simulink model "s_cd_hmc_v2"  (R2016b)
(part 14 of 43)

  Relational5/1 -> Delay3/1, Register10/2, Register4/2, Delay5/1
  Counter9/1 -> Register10/1
  Counter7/1 -> Register4/1
  pipeline155/1(q) -> data_out_counter/1(out_counter)
  pipeline156/1(q) -> data_in_counter/1(out_counter)
  Counter6/1 -> Relational5/1
  pipeline159/1(q) -> Gateway Out3/1, [radd]
  pipeline162/1(q) -> Gateway Out91/1, [din]
  pipeline163/1(q) -> Delay81/1
  [hmc_dvalid] -> Reorder_cntrl/3(dvalid)
  pipeline167/1(q) -> Gateway Out46/1, hmc/7
  pipeline168/1(q) -> Gateway Out47/1, hmc/8
  pipeline169/1(q) -> Gateway Out49/1, hmc/9
  pipeline170/1(q) -> Gateway Out51/1, hmc/10
  pipeline171/1(q) -> Gateway Out52/1, hmc/11
  pipeline172/1(q) -> Gateway Out53/1, hmc/12
  bus_expand12/1(msb_out8) -> Gateway Out40/1
  bus_expand12/5(out4) -> Gateway Out61/1
  bus_expand12/6(out3) -> Gateway Out62/1
  bus_expand12/7(out2) -> Gateway Out63/1
  bus_expand12/4(out5) -> Gateway Out60/1
  bus_expand12/3(out6) -> Gateway Out44/1
  bus_expand12/2(out7) -> Gateway Out41/1
  bus_expand12/8(lsb_out1) -> Gateway Out64/1
  bus_expand11/1(msb_out8) -> Gateway Out65/1
  bus_expand11/2(out7) -> Gateway Out66/1
  bus_expand11/3(out6) -> Gateway Out67/1
  bus_expand11/4(out5) -> Gateway Out68/1
  bus_expand11/5(out4) -> Gateway Out69/1
  bus_expand11/6(out3) -> Gateway Out70/1
  bus_expand11/7(out2) -> Gateway Out71/1
  bus_expand11/8(lsb_out1) -> Gateway Out72/1
  Gateway Out72/1 -> To Workspace66/1
  Gateway Out71/1 -> To Workspace65/1
  Gateway Out70/1 -> To Workspace64/1
  Gateway Out69/1 -> To Workspace63/1
  Gateway Out68/1 -> To Workspace62/1
  Gateway Out67/1 -> To Workspace61/1
  Gateway Out66/1 -> To Workspace35/1
  Gateway Out65/1 -> To Workspace60/1
  Gateway Out63/1 -> To Workspace58/1
  Gateway Out64/1 -> To Workspace59/1
  Gateway Out62/1 -> To Workspace57/1
  Gateway Out61/1 -> To Workspace56/1
  Gateway Out60/1 -> To Workspace55/1
  Gateway Out44/1 -> To Workspace54/1
  Gateway Out41/1 -> To Workspace53/1
  Gateway Out40/1 -> To Workspace34/1
  bus_expand13/2(out7) -> Gateway Out73/1
  bus_expand13/3(out6) -> Gateway Out74/1
  bus_expand13/4(out5) -> Gateway Out75/1
  bus_expand13/5(out4) -> Gateway Out76/1
  bus_expand13/6(out3) -> Gateway Out77/1
  bus_expand13/7(out2) -> Gateway Out78/1
  bus_expand13/8(lsb_out1) -> Gateway Out79/1
  Gateway Out79/1 -> To Workspace74/1
  Gateway Out78/1 -> To Workspace73/1
  Gateway Out77/1 -> To Workspace72/1
  Gateway Out76/1 -> To Workspace71/1
  Gateway Out75/1 -> To Workspace70/1
  Gateway Out74/1 -> To Workspace69/1
  Gateway Out73/1 -> To Workspace67/1
  [q_out] -> bus_expand13/1(bus_in)
  bus_expand13/1(msb_out8) -> Gateway Out80/1
  Gateway Out80/1 -> To Workspace68/1
  [hmc_reord_dvalid] -> FIFO1/2, Gateway Out16/1
  bus_expand1/1(msb_out8) -> pipeline37/1(d)  "hmc_out1"
  bus_expand1/8(lsb_out1) -> pipeline44/1(d)  "hmc_out8"
  [fifo1_dout] -> pipeline49/1(d)
  bus_expand2/1(msb_out8) -> pipeline26/1(d)  "hmc_out9"
  bus_expand2/8(lsb_out1) -> pipeline36/1(d)  "hmc_out16"
  [fifo0_dout] -> pipeline71/1(d)
  pipeline37/1(q) -> fifo1/1(in_d00)
  pipeline38/1(q) -> fifo1/2(in_d01)
  pipeline39/1(q) -> fifo1/3(in_d02)
  pipeline41/1(q) -> fifo1/5(in_d04)
  pipeline42/1(q) -> fifo1/6(in_d05)
  pipeline43/1(q) -> fifo1/7(in_d06)
  pipeline36/1(q) -> fifo0/8(in_d07)
  pipeline35/1(q) -> fifo0/7(in_d06)
  pipeline34/1(q) -> fifo0/6(in_d05)
  pipeline33/1(q) -> fifo0/5(in_d04)
  pipeline32/1(q) -> fifo0/4(in_d03)
  pipeline31/1(q) -> fifo0/3(in_d02)
  pipeline30/1(q) -> fifo0/2(in_d01)
  pipeline26/1(q) -> fifo0/1(in_d00)
  bus_expand1/2(out7) -> pipeline38/1(d)
  bus_expand1/4(out5) -> pipeline40/1(d)
  bus_expand1/7(out2) -> pipeline43/1(d)
  bus_expand1/3(out6) -> pipeline39/1(d)
  bus_expand2/7(out2) -> pipeline35/1(d)
  bus_expand1/5(out4) -> pipeline41/1(d)
  bus_expand1/6(out3) -> pipeline42/1(d)
  bus_expand2/5(out4) -> pipeline33/1(d)
  bus_expand2/4(out5) -> pipeline32/1(d)
  bus_expand2/6(out3) -> pipeline34/1(d)
  bus_expand2/3(out6) -> pipeline31/1(d)
  bus_expand2/2(out7) -> pipeline30/1(d)
  Convert28/1 -> pipeline45/1(d)
  pipeline44/1(q) -> fifo1/8(in_d07)
  pipeline40/1(q) -> fifo1/4(in_d03)
  Convert22/1 -> pipeline57/1(d)
  [hmc_reord_sync] -> pipeline52/1(d)
  pipeline56/1(q) -> fifo0/17(trig)
  pipeline57/1(q) -> fifo0/16(we)
  pipeline59/1(q) -> fifo0/10(in_per_full)
  pipeline58/1(q) -> fifo0/11(in_full)
  pipeline60/1(q) -> fifo0/9(in_empty)
  FIFO0/3 -> [fifo0_per_full]
  [fifo0_empty] -> pipeline64/1(d)
  [fifo0_per_full] -> pipeline63/1(d)
  [fifo0_full] -> pipeline62/1(d)
  FIFO1/3 -> [fifo1_per_full]
  [fifo0_dout] -> bus_expand12/1(bus_in)
  [fifo1_dout] -> bus_expand11/1(bus_in)
  [mux_sel] -> Gateway Out18/1, Mux/1
  pipeline45/1(q) -> fifo1/16(we)
  pipeline46/1(q) -> fifo1/17(trig)
  pipeline65/1(q) -> fifo1/9(in_empty)
  pipeline66/1(q) -> fifo1/10(in_per_full)
  pipeline67/1(q) -> fifo1/11(in_full)
  [fifo1_full] -> pipeline68/1(d)
  [fifo1_per_full] -> pipeline51/1(d)
  [fifo1_empty] -> pipeline50/1(d)
  [mux_sel] -> pipeline55/1(d)
  pipeline72/1(q) -> fifo0/12(in_mux_sel)
  pipeline73/1(q) -> fifo1/12(in_mux_sel)
  [mux_sel] -> pipeline69/1(d)
  [hmc_reord_dvalid] -> FIFO0/2, Gateway Out12/1
  Logical18/1 -> Gateway Out120/1, Delay7/1, edge_detect11/1(in)
  Convert19/1 -> Gateway Out45/1, Logical2/2
  [fifo0_dout] -> Slice11/1
  [fifo1_dout] -> Slice3/1
  Convert17/1 -> Gateway Out43/1, Logical2/1
  Counter/1 -> Convert12/1, Convert14/1
  Logical21/1 -> Gateway Out145/1, edge_detect10/1(in)
  Logical23/1 -> Gateway Out146/1, edge_detect28/1(in)
  Inverter7/1 -> Gateway Out148/1, Logical21/2
  Inverter8/1 -> Gateway Out147/1, Logical23/2
  [fifo1_re] -> FIFO1/3, Gateway Out17/1
  Convert15/1 -> Gateway Out149/1, Logical23/1
  hmc_delay/1(sim_out) -> To Workspace5/1
  [hmc_delay] -> Convert4/1
  Convert4/1 -> hmc_delay/1(out_delay)
  [hmc_sync] -> Reorder_cntrl/1(rst)
  Gateway Out22/1 -> To Workspace9/1
  Slice8/1 -> bus_expand4/1(bus_in)
  [hmc_reord_data] -> Slice8/1
  bus_expand4/1(msb_out8) -> Gateway Out22/1
  Gateway Out24/1 -> To Workspace11/1
  Gateway Out25/1 -> To Workspace18/1
  Gateway Out26/1 -> To Workspace19/1
  bus_expand4/4(out5) -> Gateway Out26/1
  bus_expand4/3(out6) -> Gateway Out25/1
  bus_expand4/2(out7) -> Gateway Out24/1
  Gateway Out27/1 -> To Workspace21/1
  bus_expand4/5(out4) -> Gateway Out27/1
  Gateway Out28/1 -> To Workspace22/1
  bus_expand4/6(out3) -> Gateway Out28/1
  Gateway Out29/1 -> To Workspace23/1
  bus_expand4/7(out2) -> Gateway Out29/1
  Gateway Out30/1 -> To Workspace24/1
  bus_expand4/8(lsb_out1) -> Gateway Out30/1
  Slice10/1 -> bus_expand6/1(bus_in)
  [hmc_reord_data] -> Slice10/1
  Gateway Out31/1 -> To Workspace77/1
  Gateway Out32/1 -> To Workspace27/1
  Gateway Out33/1 -> To Workspace28/1
  Gateway Out35/1 -> To Workspace29/1
  Gateway Out37/1 -> To Workspace31/1
  Gateway Out38/1 -> To Workspace32/1
  Gateway Out39/1 -> To Workspace33/1
  Gateway Out42/1 -> To Workspace36/1
  bus_expand6/1(msb_out8) -> Gateway Out31/1
  bus_expand6/2(out7) -> Gateway Out32/1
  bus_expand6/3(out6) -> Gateway Out33/1
  bus_expand6/4(out5) -> Gateway Out35/1
  bus_expand6/5(out4) -> Gateway Out37/1
  bus_expand6/6(out3) -> Gateway Out38/1
  bus_expand6/7(out2) -> Gateway Out39/1
  bus_expand6/8(lsb_out1) -> Gateway Out42/1
  Gateway Out99/1 -> To Workspace94/1
  Gateway Out100/1 -> To Workspace95/1
  Gateway Out101/1 -> To Workspace96/1
  Gateway Out102/1 -> To Workspace97/1
  Gateway Out103/1 -> To Workspace98/1
  cd_hmc_sync_in/1(sim_out) -> To Workspace102/1
  cd_hmc_sync_out/1(sim_out) -> To Workspace101/1
  pipeline81/1(q) -> Register1/3, Register1/1
  pipeline82/1(q) -> Register5/3, Register5/1
  Register5/1 -> pipeline132/1(d)
  pipeline102/1(q) -> Register1/2
  pipeline108/1(q) -> Register5/2
  cd_hmc_sync_in_cnt/1(sim_out) -> To Workspace104/1
  Counter10/1 -> pipeline129/1(d)
  cd_hmc_sync_out_cnt/1(sim_out) -> To Workspace105/1
  Counter11/1 -> pipeline113/1(d)
  pipeline113/1(q) -> cd_hmc_sync_out_cnt/1(out_reg)
  pipeline129/1(q) -> cd_hmc_sync_in_cnt/1(out_reg)
  pipeline131/1(q) -> cd_hmc_sync_in/1(out_reg)
  pipeline132/1(q) -> cd_hmc_sync_out/1(out_reg)
  pipeline146/1(q) -> cd_hmc_rd_tag_err_count/1(out_counter)
  pipeline147/1(q) -> cd_hmc_fifo_full/1(out_full)
  pipeline148/1(q) -> cd_hmc_fifo_empty/1(out_empty)
  [fifo1_per_full] -> pipeline14/1(d)
  pipeline165/1(q) -> cd_hmc_rd_tag_err/1(out_error)
  Register1/1 -> pipeline131/1(d)
  sync_mon_rst/1(in_reg) -> pipeline98/1(d)
  Constant18/1 -> sync_mon_rst/1(sim_1)
  pipeline91/1(q) -> Counter11/1
  pipeline110/1(q) -> Counter11/2
  pipeline90/1(q) -> Counter10/1
  pipeline109/1(q) -> Counter10/2
  Gateway Out19/1 -> To Workspace4/1
  pipeline3/1(q) -> hmc/2, Gateway Out99/1  "hmc_wadd"
  hmc/1 -> Slice42/1, Slice43/1, pipeline19/1(d), Slice6/1, Slice13/1
  Slice13/1 -> Convert16/1
  Gateway Out87/1 -> To Workspace82/1
  [hmc_win_p0] -> pipeline173/1(d)
  Gateway Out90/1 -> To Workspace85/1
  read_tag_check/1(rd_tag_err) -> pipeline165/1(d)
  read_tag_check/2(rd_tag_err_count) -> pipeline146/1(d)
  cd_hmc_wr_req_count/1(sim_out) -> To Workspace115/1
  Counter3/1 -> pipeline4/1(d)
  pipeline4/1(q) -> cd_hmc_wr_req_count/1(out_reg)
  pipeline18/1(q) -> Counter3/1
  pipeline166/1(q) -> Counter3/2
  cd_hmc_rd_req_count/1(sim_out) -> To Workspace116/1
  Counter12/1 -> pipeline177/1(d)
  pipeline177/1(q) -> cd_hmc_rd_req_count/1(out_reg)
  pipeline176/1(q) -> Counter12/1
  pipeline175/1(q) -> Counter12/2
  [hmc_dvalid] -> pipeline183/1(d)  "tp2"
  [hmc_tag_out] -> pipeline180/1(d)  "tp1"
  [hmc_tag_pol0] -> pipeline181/1(d)
  [hmc_sync] -> pipeline182/1(d)
  pipeline181/1(q) -> read_tag_check/1(HMC_tag_in)
  pipeline180/1(q) -> read_tag_check/2(HMC_tag_out)
  pipeline183/1(q) -> read_tag_check/3(HMC_dvalid)
  pipeline182/1(q) -> read_tag_check/4(HMC_sync)
  cd_hmc_rd_dvalid_count/1(sim_out) -> To Workspace119/1
  Counter13/1 -> pipeline186/1(d)
  pipeline186/1(q) -> cd_hmc_rd_dvalid_count/1(out_reg)
  pipeline185/1(q) -> Counter13/1
  pipeline184/1(q) -> Counter13/2
  Constant20/1 -> dvalid_capture_cntrl/1(sim_1)
  dvalid_capture_cntrl/1(in_reg) -> pipeline78/1(d)
  Logical15/1 -> pipeline184/1(d)
  [hmc_dvalid] -> pipeline220/1(d)
  Logical/1 -> pipeline175/1(d)
  [hmc_rin_pol0] -> pipeline217/1(d)
  Logical16/1 -> pipeline166/1(d)
  [hmc_win_pol0] -> pipeline214/1(d)
  pipeline76/1(q) -> Logical16/1
  pipeline77/1(q) -> Logical/1
  pipeline75/1(q) -> Logical15/1
  pipeline78/1(q) -> [capture_cntrl]
  [capture_cntrl] -> pipeline75/1(d)
  [capture_cntrl] -> pipeline77/1(d)
  [capture_cntrl] -> pipeline76/1(d)
  pipeline83/1(q) -> read_tag_check/5(Capture_cntrl)
  [capture_cntrl] -> pipeline83/1(d)
  pipeline213/1(q) -> pipeline18/1(d)
  Logical30/1 -> pipeline185/1(d)
  pipeline216/1(q) -> pipeline176/1(d)
  [hmc_sync] -> pipeline218/1(d)
  Constant22/1 -> dvalid_capture_cntrl_rst/1(sim_1)
  dvalid_capture_cntrl_rst/1(in_reg) -> pipeline84/1(d)
  pipeline84/1(q) -> edge_detect16/1
  [capture_cntrl_rst] -> pipeline216/1(d)
  [capture_cntrl_rst] -> pipeline219/1(d)
  [capture_cntrl_rst] -> pipeline213/1(d)
  cd_reord_sync_out/1(sim_out) -> To Workspace117/1
  Register12/1 -> pipeline85/1(d)
  [sync_mon_rst] -> edge_detect1/1
  pipeline85/1(q) -> cd_reord_sync_out/1(out_reg)
  pipeline86/1(q) -> Register12/3, Register12/1
  [sync_mon_rst] -> edge_detect31/1
  pipeline98/1(q) -> [sync_mon_rst]
  cd_reord_sync_cnt/1(sim_out) -> To Workspace118/1
  Counter14/1 -> pipeline88/1(d)
  pipeline88/1(q) -> cd_reord_sync_cnt/1(out_reg)
  pipeline87/1(q) -> Counter14/2
  pipeline92/1(q) -> Register12/2
  pipeline89/1(q) -> Counter14/1
  [hmc_rin_p0] -> pipeline17/1(d)
  [hmc_raddr_p0] -> pipeline5/1(d)
  [hmc_tag_p0] -> pipeline16/1(d)
  cd_hmc_sync/1(sim_out) -> To Workspace112/1
  Counter15/1 -> pipeline95/1(d)
  pipeline95/1(q) -> cd_hmc_sync/1(out_reg)
  pipeline94/1(q) -> Counter15/1
  pipeline93/1(q) -> Counter15/2
  [hmc_sync] -> pipeline211/1(d)
  [sync_mon_rst] -> pipeline210/1(d)
  pipeline210/1(q) -> edge_detect23/1
  pipeline211/1(q) -> edge_detect17/1
  Logical35/1 -> Counter1/2, Gateway Out8/1
  [hmc_dout] -> HMC_reord_bram/2, Gateway Out11/1, Slice33/1, Slice32/1
  Gateway Out98/1 -> To Workspace100/1
  Gateway Out105/1 -> To Workspace109/1
  hmc/2 -> Logical34/2, pipeline20/1(d), Gateway Out105/1
  [wadd] -> hmc_control/1(waddr)
  [hmc_delay] -> hmc_control/2(delay)
  [hmc_sync] -> hmc_control/3(sync_in)
  [win] -> hmc_control/4(win)
  [rin] -> hmc_control/5(rin)
  [radd] -> hmc_control/6(rdadd)
  [din] -> hmc_control/7(din)
  hmc_control/3(hmc_rin) -> [hmc_rin_pol0]
  hmc_control/4(hmc_raddr) -> [hmc_raddr_pol0]
  hmc_control/6(hmc_tag) -> [hmc_tag_pol0]
  [hmc_rin_pol0] -> pipeline198/1(d)
  [hmc_tag_out] -> pipeline193/1(d)
  [hmc_tag_pol0] -> pipeline196/1(d)
  [hmc_raddr_pol0] -> pipeline197/1(d)
  [hmc_rd_rdy] -> pipeline194/1(d)
  [hmc_dvalid] -> pipeline195/1(d)
  pipeline6/1(q) -> hmc_debug0_p0/4(in_rin)
  pipeline7/1(q) -> hmc_debug0_p0/5(in_rdaddr)
  pipeline8/1(q) -> hmc_debug0_p0/6(in_tag_in)
  pipeline96/1(q) -> hmc_debug0_p0/7(in_dvalid)
  pipeline99/1(q) -> hmc_debug0_p0/8(in_rd_rdy)
  pipeline100/1(q) -> hmc_debug0_p0/9(in_tag_out)
  pipeline178/1(q) -> Gateway Out57/1, hmc_debug0_p0/10(we)
  [hmc_tag_out] -> pipeline188/1(d)
  [hmc_rd_rdy] -> pipeline189/1(d)
  [hmc_dvalid] -> pipeline190/1(d)
  pipeline191/1(q) -> hmc_debug1_p0/1(in_dvalid)
  pipeline192/1(q) -> hmc_debug1_p0/2(in_rd_rdy)
  pipeline179/1(q) -> hmc_debug1_p0/3(in_tag_out)
  pipeline187/1(q) -> hmc_debug1_p0/4(we)
  pipeline188/1(q) -> pipeline179/1(d)
  pipeline189/1(q) -> pipeline192/1(d)
  pipeline190/1(q) -> pipeline191/1(d)
  pipeline193/1(q) -> pipeline100/1(d)
  pipeline194/1(q) -> pipeline99/1(d)
  pipeline195/1(q) -> pipeline96/1(d)
  pipeline196/1(q) -> pipeline8/1(d)
  pipeline197/1(q) -> pipeline7/1(d)
  pipeline198/1(q) -> pipeline6/1(d)
  pipeline199/1(q) -> [rin], Gateway Out4/1
  [hmc_wr_ready] -> pipeline200/1(d)
  pipeline200/1(q) -> pipeline201/1(d)
  pipeline201/1(q) -> hmc_debug0_p0/2(in_wr_rdy)
  [hmc_win_pol0] -> pipeline203/1(d)
  [hmc_waddr_pol0] -> pipeline202/1(d)
  pipeline202/1(q) -> pipeline204/1(d)
  pipeline203/1(q) -> pipeline205/1(d)
  pipeline204/1(q) -> Gateway Out58/1, hmc_debug0_p0/3(in_waddr)
  pipeline205/1(q) -> Gateway Out59/1, hmc_debug0_p0/1(in_win)
  Delay28/1 -> Delay31/1
  Gateway Out1/1 -> To Workspace6/1
  Gateway Out2/1 -> To Workspace7/1
  Gateway Out3/1 -> To Workspace8/1
  Gateway Out4/1 -> To Workspace20/1
  Convert2/1 -> Delay22/1, addr/2
  pipeline214/1(q) -> Logical16/2
  pipeline217/1(q) -> Logical/2
  pipeline218/1(q) -> Logical30/1
  pipeline219/1(q) -> Logical30/2
  pipeline220/1(q) -> Logical15/2
  Logical24/1 -> addr/1, addr_stall/1
  pipeline13/1(q) -> Logical24/1
  pipeline9/1(q) -> Logical27/1
  edge_detect24/1(out) -> Logical24/2
  pipeline2/1(q) -> [hmc_delay]
  pipeline206/1(q) -> [dout]
  pipeline12/1(q) -> Delay23/1
  pipeline157/1(q) -> Gateway Out86/1, hmc_debug0_p0/11(trig)
  Logical32/1 -> edge_detect13/1(in)
  Logical29/1 -> edge_detect5/1(in)
  pipeline158/1(q) -> hmc_debug1_p0/5(trig)
  Delay36/1 -> Delay33/1
  pipeline23/1(q) -> [hmc_rd_rdy]  "rd_ready"
  AddSub/1 -> Delay32/1  "rd_add_HR"
  Gateway Out5/1 -> To Workspace30/1
  Gateway Out6/1 -> To Workspace75/1
  Reorder_cntrl/1(bram_rd_addr) -> Gateway Out6/1, HMC_reord_bram/4
  Gateway Out7/1 -> To Workspace76/1
  [hmc_tag_out] -> Reorder_cntrl/2(tag)
  Gateway Out13/1 -> To Workspace84/1
  Gateway Out11/1 -> To Workspace81/1
  pipeline209/1(q) -> [hmc_sync], Gateway Out19/1
  Slice18/1 -> Convert20/1
  [hmc_dvalid] -> Gateway Out13/1, HMC_reord_bram/3
  Convert1/1 -> [hmc_dvalid]
  pipeline1/1(q) -> Delay37/1
  pipeline79/1(q) -> [q_dvalid], Gateway Out84/1, dv/1
  Slice19/1 -> Convert21/1
  [hmc_sync] -> Counter1/1
  edge_detect11/1(out) -> Gateway Out142/1
  Logical4/1 -> Convert15/1
  Inverter1/1 -> Gateway Out150/1, Logical4/1
  Delay7/1 -> Counter/2, Gateway Out143/1, Logical4/2
  Convert12/1 -> Inverter1/1
  hmc_wr_err/1(sim_out) -> To Workspace136/1
  Counter16/1 -> pipeline10/1(d)
  pipeline10/1(q) -> hmc_wr_err/1(out_reg)
  pipeline223/1(q) -> Counter16/1
  [sync_mon_rst] -> edge_detect26/1
  [hmc_wr_ready] -> Inverter/1
  Inverter/1 -> Logical5/1
  pipeline224/1(q) -> Counter16/2
  Logical5/1 -> pipeline224/1(d)
  hmc_rd_err/1(sim_out) -> To Workspace137/1
  Counter17/1 -> pipeline225/1(d)
  pipeline225/1(q) -> hmc_rd_err/1(out_reg)
  pipeline226/1(q) -> Counter17/1
  [sync_mon_rst] -> edge_detect15/1
  [hmc_rd_rdy] -> Inverter12/1
  Inverter12/1 -> Logical6/1
  pipeline227/1(q) -> Counter17/2
  Logical6/1 -> pipeline227/1(d)
  [hmc_rd_rdy] -> Logical31/1
  Logical31/1 -> edge_detect24/1(in), Logical27/2
  Delay33/1 -> pipeline209/1(d)
  Delay32/1 -> pipeline159/1(d)
  Delay31/1 -> pipeline232/1(d), pipeline199/1(d)
  Delay25/1 -> pipeline162/1(d)
  [hmc_reord_data] -> Slice17/1
  [hmc_reord_data] -> Slice20/1
  Slice21/1 -> Convert17/1
  Slice22/1 -> Convert19/1
  [fifo0_dout] -> Slice21/1
  [fifo1_dout] -> Slice22/1
  Gateway Out8/1 -> To Workspace78/1
  Gateway Out9/1 -> To Workspace79/1
  Gateway Out10/1 -> To Workspace80/1
  Gateway Out12/1 -> To Workspace83/1
  Gateway Out14/1 -> To Workspace86/1
  [fifo0_re] -> FIFO0/3, Gateway Out14/1
  Gateway Out15/1 -> To Workspace87/1
  Gateway Out16/1 -> To Workspace88/1
  Gateway Out17/1 -> To Workspace89/1
  Gateway Out20/1 -> To Workspace91/1
  Gateway Out21/1 -> To Workspace92/1
  [hmc_reord_sync] -> pipeline86/1(d), pipeline87/1(d)
  Gateway Out18/1 -> To Workspace90/1
  Gateway Out36/1 -> To Workspace106/1
  Gateway Out81/1 -> To Workspace107/1
  Slice24/1 -> Convert23/1
  Convert24/1 -> Logical33/2
  Convert23/1 -> Logical33/1
  Slice25/1 -> Convert24/1
  Logical33/1 -> Convert25/1
  Convert25/1 -> edge_detect32/1
  [fifo_sync] -> delay1/1  "sync"
  Gateway Out82/1 -> To Workspace108/1
  HMC_reord_bram/2 -> Delay2/1, Slice25/1, Slice24/1, Slice18/1, Slice19/1
  Gateway Out23/1 -> To Workspace93/1
  Gateway Out34/1 -> To Workspace99/1
  Gateway Out83/1 -> To Workspace110/1
  Gateway Out84/1 -> To Workspace111/1
  Gateway Out85/1 -> To Workspace113/1
  [fifo_dvalid] -> delay8/1
  Counter19/1 -> Convert29/1
  Convert29/1 -> [mux_sel]
  [hmc_sync] -> Counter19/1
  Gateway Out43/1 -> To Workspace37/1
  Gateway Out45/1 -> To Workspace38/1
  Logical27/1 -> addr_stall/2
  misci/1 -> Gateway Out138/1, Slice29/1, Delay21/1
  [sync_in] -> pipeline1/1(d), pipeline13/1(d)
  [en_in] -> pipeline9/1(d), pipeline12/1(d)
  en/1 -> Gateway Out140/1, [en_in]  "en_in"
  Delay70/1 -> pipeline233/1(d)
  AddSub2/1 -> AddSub/2
  Constant/1 -> AddSub2/2
  [delay_in] -> AddSub2/1
  Slice29/1 -> [ld_val]
  pipeline232/1(q) -> Gateway Out2/1, [win]
  [hmc_tag_out] -> Gateway Out5/1, HMC_reord_bram/1
  [ld_val] -> Register13/2
  delay/1 -> Register13/1  "delay"
  Register13/1 -> [delay_in], pipeline2/1(d)
  hmc_wr_rd_rdy_clash/1(sim_out) -> To Workspace124/1
  Counter20/1 -> pipeline207/1(d)
  pipeline207/1(q) -> hmc_wr_rd_rdy_clash/1(out_reg)
  pipeline208/1(q) -> Counter20/1
  pipeline231/1(q) -> Counter20/2
  [sync_mon_rst] -> edge_detect14/1
  [hmc_rd_rdy] -> Logical19/2
  [hmc_wr_ready] -> Logical19/1
  Logical19/1 -> pipeline231/1(d)
  Gateway Out91/1 -> To Workspace125/1
  Gateway Out93/1 -> To Workspace126/1
  delay2/1 -> Terminator1/1, Gateway Out34/1
  Gateway Out106/1 -> To Workspace132/1
  Gateway Out107/1 -> To Workspace133/1
  Gateway Out108/1 -> To Workspace134/1
  pipeline233/1(q) -> Gateway Out1/1, [wadd]
  Delay1/1 -> Delay70/1
  delay1/1 -> pipeline117/1(d), Gateway Out108/1
  delay8/1 -> pipeline79/1(d), Gateway Out107/1
  Slice5/1 -> Convert7/1
  Gateway Out121/1 -> To Workspace150/1
  Convert7/1 -> Gateway Out121/1
  Convert20/1 -> Logical35/1
  Convert21/1 -> Logical35/2
  Delay2/1 -> Gateway Out93/1, [hmc_reord_data]
  Convert8/1 -> [hmc_reord_dvalid], Gateway Out9/1
  [hmc_waddr_p0] -> pipeline3/1(d)
  Gateway Out50/1 -> To Workspace43/1
  delay4/1 -> Gateway Out23/1, [fifo_sync]
  [fifo0_per_full] -> pipeline151/1(d)
  pipeline14/1(q) -> cd_hmc_fifo1_level/1(out_level)
  pipeline151/1(q) -> cd_hmc_fifo0_level/1(out_level)
  [sync_mon_rst] -> edge_detect18/1
  edge_detect31/1 -> pipeline102/1(d), pipeline90/1(d)
  edge_detect12/1 -> pipeline109/1(d), pipeline81/1(d)
  edge_detect18/1 -> pipeline108/1(d), pipeline91/1(d)
  edge_detect20/1 -> pipeline82/1(d), pipeline110/1(d)
  edge_detect32/1 -> Delay8/1
  Counter1/1 -> Convert8/1
  edge_detect1/1 -> pipeline89/1(d), pipeline92/1(d)
  edge_detect15/1 -> pipeline226/1(d)
  edge_detect26/1 -> pipeline223/1(d)
  edge_detect14/1 -> pipeline208/1(d)
  edge_detect7/1 -> [sync_trig]
  edge_detect16/1 -> [capture_cntrl_rst]
  edge_detect13/1(out) -> pipeline160/1(d), pipeline161/1(d), pipeline157/1(d)
  edge_detect23/1 -> pipeline94/1(d)
  edge_detect17/1 -> pipeline93/1(d)
  edge_detect2/1 -> Counter2/1
  edge_detect4/1 -> Counter4/1
  Delay3/1 -> Counter9/1
  Delay5/1 -> Counter7/1
  Slice6/1 -> Convert30/1
  Convert30/1 -> Logical20/1
  Convert16/1 -> Logical20/2
  Slice9/1 -> Convert11/1
  Slice12/1 -> Convert31/1
  Convert31/1 -> Logical28/1
  Convert11/1 -> Logical28/2
  Logical28/1 -> edge_detect12/1, Gateway Out90/1
  Slice27/1 -> Convert32/1
  Slice16/1 -> Convert33/1
  Convert33/1 -> Logical29/1
  Convert32/1 -> Logical29/2
  [hmc_dout] -> Slice27/1, Slice16/1
  Slice2/1 -> Convert5/1
  Slice1/1 -> Convert6/1
  Convert6/1 -> Logical32/1
  Convert5/1 -> Logical32/2
  [hmc_din_pol0] -> Slice2/1, Slice1/1
  Delay6/1 -> Delay13/1
  [hmc_post] -> Logical31/3
  [hmc_init] -> Logical31/2
  FIFO0/1 -> [fifo0_dout], Gateway Out50/1
  FIFO1/1 -> [fifo1_dout]
  Slice3/1 -> Mux/3, Gateway Out81/1
  Slice11/1 -> Gateway Out36/1, Mux/2
  Delay8/1 -> Gateway Out82/1, [hmc_reord_sync]
  [hmc_win_p1] -> pipeline167/1(d)
  [hmc_waddr_p1] -> pipeline168/1(d)
  [hmc_din_p1] -> pipeline169/1(d)
  [hmc_rin_p1] -> pipeline170/1(d)
  [hmc_raddr_p1] -> pipeline171/1(d)
  [hmc_tag_p1] -> pipeline172/1(d)
  hmc/7 -> Gateway Out56/1, pipeline61/1(d)
  hmc/6 -> Gateway Out55/1, pipeline11/1(d)
  hmc/8 -> pipeline152/1(d)
  hmc/9 -> pipeline153/1(d)
  hmc/10 -> Gateway Out54/1, pipeline154/1(d)
  pipeline154/1(q) -> [hmc_tag_out_pol1]
  pipeline153/1(q) -> [hmc_rd_rdy_pol1]
  pipeline152/1(q) -> [hmc_wr_rdy_pol1]
  pipeline61/1(q) -> [hmc_dvalid_pol1]
  pipeline11/1(q) -> [hmc_dout_pol1]
  [hmc_din_p0] -> pipeline174/1(d)
  Register14/1 -> pipeline260/1(d), pipeline271/1(d), pipeline178/1(d)
  [hmc_win_pol0] -> Register14/3, Register14/1
  [sync_mon_rst] -> edge_detect19/1(in)
  [hmc_dvalid] -> Register15/3, Register15/1
  [sync_mon_rst] -> edge_detect21/1(in)
  edge_detect19/1(out) -> Register14/2
  edge_detect21/1(out) -> Register15/2
  Gateway Out46/1 -> To Workspace39/1
  Gateway Out47/1 -> To Workspace40/1
  Gateway Out49/1 -> To Workspace42/1
  Gateway Out51/1 -> To Workspace44/1
  Gateway Out52/1 -> To Workspace45/1
  Gateway Out53/1 -> To Workspace46/1
  Gateway Out54/1 -> To Workspace47/1
  Gateway Out55/1 -> To Workspace48/1
  Gateway Out56/1 -> To Workspace49/1
  bus_expand3/1(msb_out8) -> pipeline252/1(d)  "hmc_out1"
  bus_expand3/8(lsb_out1) -> pipeline259/1(d)  "hmc_out8"
  Slice28/1 -> bus_expand3/1(bus_in)
  bus_expand7/1(msb_out8) -> pipeline244/1(d)  "hmc_out9"
  bus_expand7/8(lsb_out1) -> pipeline251/1(d)  "hmc_out16"
  Slice30/1 -> bus_expand7/1(bus_in)
  pipeline252/1(q) -> hmc_din0_p0/1(in_d00)
  pipeline253/1(q) -> Gateway Out94/1, hmc_din0_p0/2(in_d01)
  pipeline254/1(q) -> hmc_din0_p0/3(in_d02)
  pipeline256/1(q) -> hmc_din0_p0/5(in_d04)
  pipeline257/1(q) -> hmc_din0_p0/6(in_d05)
  pipeline258/1(q) -> hmc_din0_p0/7(in_d06)
  pipeline260/1(q) -> hmc_din0_p0/9(we)
  pipeline160/1(q) -> hmc_din0_p0/10(trig)
  pipeline251/1(q) -> Gateway Out92/1, hmc_din1_p0/8(in_d07)
  pipeline250/1(q) -> hmc_din1_p0/7(in_d06)
  pipeline249/1(q) -> hmc_din1_p0/6(in_d05)
  pipeline248/1(q) -> hmc_din1_p0/5(in_d04)
  pipeline247/1(q) -> hmc_din1_p0/4(in_d03)
  pipeline246/1(q) -> hmc_din1_p0/3(in_d02)
  pipeline245/1(q) -> Gateway Out89/1, hmc_din1_p0/2(in_d01)
  pipeline244/1(q) -> hmc_din1_p0/1(in_d00)
  bus_expand3/2(out7) -> pipeline253/1(d)
  bus_expand3/4(out5) -> pipeline255/1(d)
  bus_expand3/7(out2) -> pipeline258/1(d)
  bus_expand3/3(out6) -> pipeline254/1(d)
  bus_expand7/7(out2) -> pipeline250/1(d)
  bus_expand3/5(out4) -> pipeline256/1(d)
  bus_expand3/6(out3) -> pipeline257/1(d)
  bus_expand7/5(out4) -> pipeline248/1(d)
  bus_expand7/4(out5) -> pipeline247/1(d)
  bus_expand7/6(out3) -> pipeline249/1(d)
  bus_expand7/3(out6) -> pipeline246/1(d)
  bus_expand7/2(out7) -> pipeline245/1(d)
  [hmc_din_pol0] -> pipeline212/1(d), pipeline164/1(d)
  pipeline164/1(q) -> Slice30/1
  pipeline259/1(q) -> Gateway Out95/1, hmc_din0_p0/8(in_d07)
  pipeline255/1(q) -> hmc_din0_p0/4(in_d03)
  pipeline271/1(q) -> hmc_din1_p0/9(we), Gateway Out88/1
  pipeline161/1(q) -> hmc_din1_p0/10(trig)
  pipeline212/1(q) -> Slice28/1
  edge_detect5/1(out) -> pipeline215/1(d), pipeline221/1(d), pipeline158/1(d)
  Register15/1 -> pipeline266/1(d), pipeline265/1(d), pipeline187/1(d)
  bus_expand9/1(msb_out8) -> pipeline240/1(d)  "hmc_out1"
  bus_expand9/8(lsb_out1) -> pipeline264/1(d)  "hmc_out8"
  Slice4/1 -> bus_expand9/1(bus_in)
  bus_expand10/1(msb_out8) -> pipeline229/1(d)  "hmc_out9"
  bus_expand10/8(lsb_out1) -> pipeline239/1(d)  "hmc_out16"
  Slice26/1 -> bus_expand10/1(bus_in)
  pipeline240/1(q) -> hmc_dout0_p0/1(in_d00)
  pipeline241/1(q) -> hmc_dout0_p0/2(in_d01)
  pipeline242/1(q) -> hmc_dout0_p0/3(in_d02)
  pipeline261/1(q) -> hmc_dout0_p0/5(in_d04)
  pipeline262/1(q) -> hmc_dout0_p0/6(in_d05)
  pipeline263/1(q) -> hmc_dout0_p0/7(in_d06)
  pipeline265/1(q) -> hmc_dout0_p0/9(we)
  pipeline215/1(q) -> hmc_dout0_p0/10(trig)
  pipeline239/1(q) -> hmc_dout1_p0/8(in_d07)
  pipeline238/1(q) -> hmc_dout1_p0/7(in_d06)
  pipeline237/1(q) -> hmc_dout1_p0/6(in_d05)
  pipeline236/1(q) -> hmc_dout1_p0/5(in_d04)
  pipeline235/1(q) -> hmc_dout1_p0/4(in_d03)
  pipeline234/1(q) -> hmc_dout1_p0/3(in_d02)
  pipeline230/1(q) -> hmc_dout1_p0/2(in_d01)
  pipeline229/1(q) -> hmc_dout1_p0/1(in_d00)
  bus_expand9/2(out7) -> pipeline241/1(d)
  bus_expand9/4(out5) -> pipeline243/1(d)
  bus_expand9/7(out2) -> pipeline263/1(d)
  bus_expand9/3(out6) -> pipeline242/1(d)
  bus_expand10/7(out2) -> pipeline238/1(d)
  bus_expand9/5(out4) -> pipeline261/1(d)
  bus_expand9/6(out3) -> pipeline262/1(d)
  bus_expand10/5(out4) -> pipeline236/1(d)
  bus_expand10/4(out5) -> pipeline235/1(d)
  bus_expand10/6(out3) -> pipeline237/1(d)
  bus_expand10/3(out6) -> pipeline234/1(d)
  bus_expand10/2(out7) -> pipeline230/1(d)
  [hmc_dout] -> pipeline222/1(d), pipeline228/1(d)
  pipeline222/1(q) -> Slice26/1
  pipeline264/1(q) -> hmc_dout0_p0/8(in_d07)
  pipeline243/1(q) -> hmc_dout0_p0/4(in_d03)
  pipeline266/1(q) -> hmc_dout1_p0/9(we)
  pipeline221/1(q) -> hmc_dout1_p0/10(trig)
  pipeline228/1(q) -> Slice4/1
  Gateway Out57/1 -> To Workspace50/1
  Gateway Out58/1 -> To Workspace51/1
  Gateway Out59/1 -> To Workspace52/1
  Gateway Out86/1 -> To Workspace114/1
  Gateway Out88/1 -> To Workspace120/1
  Gateway Out89/1 -> To Workspace121/1
  Gateway Out92/1 -> To Workspace122/1
  Gateway Out94/1 -> To Workspace123/1
  Gateway Out95/1 -> To Workspace127/1
  Delay9/1 -> Delay28/1
  addr_stall1/1 -> Slice31/1  "stall"
  Convert3/1 -> addr1/2, [hmc_clear_win]
  [hmc_init] -> Logical7/1
  [hmc_post] -> Logical7/2
  Logical7/1 -> Logical11/2, Delay11/1
  Delay11/1 -> addr_stall1/2
  [clear_hmc_addr_range] -> Shift/1
  Relational/1 -> Gateway Out97/1, Register/3, Register/1
  Register/1 -> [hmc_clear_done]
  [hmc_clear_done] -> Gateway Out96/1, Mux1/1
  [hmc_clear_done] -> Mux2/1
  [hmc_clear_wraddr_pol0] -> Mux1/2
  Mux1/1 -> Gateway Out109/1, [hmc_waddr_p0]
  hmc_control/1(hmc_wraddr) -> [hmc_waddr_pol0]
  Mux2/1 -> Gateway Out110/1, [hmc_win_p0]
  hmc_control/2(hmc_win) -> [hmc_win_pol0]
  [hmc_clear_done] -> Mux3/1
  Mux3/1 -> Gateway Out111/1, [hmc_din_p0]
  hmc_control/5(hmc_din_256) -> [hmc_din_pol0]
  Constant4/1 -> Mux3/2
  [hmc_clear_win] -> Mux2/2
  Gateway Out96/1 -> To Workspace128/1
  edge_detect22/1 -> addr_stall1/1, addr1/1, Register/2, Gateway Out116/1
  Gateway Out109/1 -> To Workspace131/1
  Gateway Out110/1 -> To Workspace135/1
  Gateway Out111/1 -> To Workspace138/1
  [hmc_clear_done] -> Mux4/1, Gateway Out115/1
  [hmc_clear_done] -> Mux5/1
  [hmc_clear_wraddr_pol1] -> Mux4/2
  [hmc_waddr_pol1] -> Mux4/3
  Mux4/1 -> [hmc_waddr_p1], Gateway Out112/1
  Mux5/1 -> [hmc_win_p1], Gateway Out113/1
  [hmc_win_pol1] -> Mux5/3
  [hmc_clear_done] -> Mux6/1
  Mux6/1 -> [hmc_din_p1], Gateway Out114/1
  [hmc_din_pol1] -> Mux6/3
  Constant5/1 -> Mux6/2
  [hmc_clear_win] -> Mux5/2
  Gateway Out115/1 -> To Workspace139/1
  Gateway Out112/1 -> To Workspace140/1
  Gateway Out113/1 -> To Workspace141/1
  Gateway Out114/1 -> To Workspace142/1
  Concat1/1 -> Gateway Out158/1, [hmc_clear_wraddr_pol1]
  Constant7/1 -> Concat1/2
  [hmc_waddr_pol0] -> Mux1/3
  [hmc_win_pol0] -> Mux2/3
  [hmc_din_pol0] -> Mux3/3
  Logical11/1 -> edge_detect22/1
  clear_hmc/1(in_reg) -> pipeline267/1(d)
  Constant8/1 -> Delay/1
  [clear_hmc] -> Logical11/1
  pipeline267/1(q) -> edge_detect25/1
  Gateway Out97/1 -> To Workspace129/1
  Gateway Out104/1 -> To Workspace130/1
  Gateway Out116/1 -> To Workspace143/1
  Delay/1 -> clear_hmc/1(sim_1)
  edge_detect25/1 -> [clear_hmc]
  Slice31/1 -> edge_detect27/1
  Gateway Out117/1 -> To Workspace144/1
  [hmc_clear_done] -> pipeline268/1(d)
  pipeline268/1(q) -> hmc_clear_done/1(out_level)
  hmc_clear_done/1(sim_out) -> To Workspace145/1
  edge_detect27/1 -> Gateway Out117/1, Convert3/1
  Logical20/1 -> Gateway Out118/1, Logical34/1
  Logical34/1 -> edge_detect20/1, Gateway Out87/1
  Gateway Out118/1 -> To Workspace146/1
  Slice32/1 -> Convert18/1
  Convert26/1 -> Logical36/2
  Convert18/1 -> Logical36/1
  Slice33/1 -> Convert26/1
  Logical36/1 -> Convert27/1
  Convert27/1 -> edge_detect3/1
  Gateway Out119/1 -> To Workspace147/1
  edge_detect3/1 -> Gateway Out119/1
  [hmc_reord_sync] -> pipeline140/1(d)
  pipeline138/1(q) -> hmc_reord1/11(we)
  pipeline144/1(q) -> hmc_reord1/12(trig)
  [hmc_reord_sync] -> pipeline74/1(d)
  [hmc_reord_dvalid] -> Register16/1, Register16/3, pipeline139/1(d)
  [sync_mon_rst] -> edge_detect6/1(in)
  edge_detect6/1(out) -> Register16/2, Register17/2
  Register16/1 -> Convert37/1
  [hmc_reord_dvalid] -> pipeline29/1(d), Register17/3, Register17/1
  [hmc_reord_sync] -> pipeline80/1(d)
  Register17/1 -> Convert36/1
  [sync_mon_rst] -> edge_detect8/1(in)
  edge_detect8/1(out) -> Register18/2
  Register18/1 -> Convert22/1
  [sync_mon_rst] -> edge_detect9/1(in)
  edge_detect9/1(out) -> Register19/2
  Register19/1 -> Convert28/1
  Convert36/1 -> pipeline138/1(d)
  Convert37/1 -> pipeline128/1(d)
  [hmc_clear_done] -> Logical31/4
  sync/1 -> Gateway Out139/1, [sync_in]  "sync_in"
  pipeline54/1(q) -> hmc_reord0/10(in_sync)
  pipeline48/1(q) -> hmc_reord0/9(in_dvalid)
  pipeline150/1(q) -> hmc_reord1/10(in_sync)
  pipeline149/1(q) -> hmc_reord1/9(in_dvalid)
  pipeline269/1(q) -> fifo0/14(in_dvalid)
  pipeline270/1(q) -> fifo0/15(in_sync)
  pipeline275/1(q) -> fifo1/15(in_sync)
  pipeline274/1(q) -> fifo1/14(in_dvalid)
  Logical9/1 -> pipeline70/1(d), Register19/1, Register19/3, pipeline53/1(d), Register18/3, Register18/1
  [hmc_win_pol0] -> Logical5/2
  [hmc_clear_done] -> Logical5/3
  [hmc_clear_done] -> Logical6/3
  [hmc_rin_pol0] -> Logical6/2
  Delay14/1 -> [hmc_tag_p0]
  [hmc_tag_pol0] -> Delay14/1
  [hmc_raddr_pol0] -> Delay12/1
  Delay12/1 -> [hmc_raddr_p0]
  [hmc_rin_pol0] -> Delay15/1
  Delay15/1 -> [hmc_rin_p0]
  [hmc_raddr_pol1] -> Delay18/1
  [hmc_tag_pol1] -> Delay19/1
  [hmc_rin_pol1] -> Delay20/1
  Delay18/1 -> [hmc_raddr_p1]
  Delay19/1 -> [hmc_tag_p1]
  Delay20/1 -> [hmc_rin_p1]
  Gateway Out48/1 -> To Workspace164/1
  Slice35/1 -> bus_expand14/1(bus_in)
  [hmc_din_p0] -> pipeline278/1(d)
  bus_expand14/1(msb_out8) -> Gateway Out48/1
  Gateway Out122/1 -> To Workspace41/1
  Gateway Out123/1 -> To Workspace149/1
  Gateway Out124/1 -> To Workspace151/1
  bus_expand14/4(out5) -> Gateway Out124/1
  bus_expand14/3(out6) -> Gateway Out123/1
  bus_expand14/2(out7) -> Gateway Out122/1
  Gateway Out125/1 -> To Workspace152/1
  bus_expand14/5(out4) -> Gateway Out125/1
  Gateway Out126/1 -> To Workspace153/1
  bus_expand14/6(out3) -> Gateway Out126/1
  Gateway Out127/1 -> To Workspace154/1
  bus_expand14/7(out2) -> Gateway Out127/1
  Gateway Out128/1 -> To Workspace155/1
  bus_expand14/8(lsb_out1) -> Gateway Out128/1
  Slice34/1 -> bus_expand15/1(bus_in)
  [hmc_din_p0] -> pipeline279/1(d)
  Gateway Out129/1 -> To Workspace156/1
  Gateway Out130/1 -> To Workspace157/1
  Gateway Out131/1 -> To Workspace158/1
  Gateway Out132/1 -> To Workspace159/1
  Gateway Out133/1 -> To Workspace160/1
  Gateway Out134/1 -> To Workspace161/1
  Gateway Out135/1 -> To Workspace162/1
  Gateway Out136/1 -> To Workspace163/1
  bus_expand15/1(msb_out8) -> Gateway Out129/1
  bus_expand15/2(out7) -> Gateway Out130/1
  bus_expand15/3(out6) -> Gateway Out131/1
  bus_expand15/4(out5) -> Gateway Out132/1
  bus_expand15/5(out4) -> Gateway Out133/1
  bus_expand15/6(out3) -> Gateway Out134/1
  bus_expand15/7(out2) -> Gateway Out135/1
  bus_expand15/8(lsb_out1) -> Gateway Out136/1
  pipeline278/1(q) -> Slice35/1
  pipeline279/1(q) -> Slice34/1
  Gateway Out137/1 -> To Workspace165/1
  Gateway Out138/1 -> To Workspace166/1
  Gateway Out139/1 -> To Workspace167/1
  Gateway Out140/1 -> To Workspace168/1
  Gateway Out141/1 -> To Workspace169/1
  Delay81/1 -> delay10/1
  Constant1/1 -> [clear_hmc_addr_range]
  pipeline27/1(q) -> bus_expand5/1(bus_in)
  pipeline28/1(q) -> bus_expand8/1(bus_in)
  pipeline29/1(q) -> pipeline149/1(d)
  pipeline80/1(q) -> pipeline150/1(d), pipeline144/1(d)
  pipeline139/1(q) -> pipeline48/1(d)
  pipeline140/1(q) -> pipeline54/1(d), pipeline137/1(d)
  pipeline52/1(q) -> pipeline56/1(d), pipeline270/1(d)
  pipeline53/1(q) -> pipeline269/1(d)
  pipeline55/1(q) -> pipeline72/1(d)
  pipeline62/1(q) -> pipeline58/1(d)
  pipeline63/1(q) -> pipeline59/1(d)
  pipeline64/1(q) -> pipeline60/1(d)
  pipeline71/1(q) -> bus_expand2/1(bus_in)
  pipeline49/1(q) -> bus_expand1/1(bus_in)
  pipeline50/1(q) -> pipeline65/1(d)
  pipeline51/1(q) -> pipeline66/1(d)
  pipeline68/1(q) -> pipeline67/1(d)
  pipeline69/1(q) -> pipeline73/1(d)
  pipeline70/1(q) -> pipeline274/1(d)
  pipeline74/1(q) -> pipeline46/1(d), pipeline275/1(d)
  Convert10/1 -> Logical9/2
  Convert9/1 -> Logical9/1
  Slice7/1 -> Convert9/1
  Slice23/1 -> Convert10/1
  [fifo0_dout] -> Slice7/1
  [fifo1_dout] -> Slice23/1
  Gateway Out120/1 -> To Workspace103/1
  Gateway Out142/1 -> To Workspace148/1
  Gateway Out143/1 -> To Workspace170/1
  Gateway Out144/1 -> To Workspace171/1
  Convert14/1 -> Gateway Out144/1, Logical21/1
  Gateway Out145/1 -> To Workspace172/1
  Gateway Out146/1 -> To Workspace173/1
  Gateway Out147/1 -> To Workspace174/1
  Gateway Out148/1 -> To Workspace175/1
  Gateway Out149/1 -> To Workspace176/1
  Gateway Out150/1 -> To Workspace177/1
  Gateway Out151/1 -> To Workspace178/1
  Gateway Out152/1 -> To Workspace179/1
  Inverter3/1 -> Gateway Out151/1, Logical18/1
  Inverter4/1 -> Gateway Out152/1, Logical18/2
  Gateway Out153/1 -> To Workspace180/1
  Gateway Out154/1 -> To Workspace181/1
  pipeline97/1(q) -> fifo0/13(in_re)
  pipeline101/1(q) -> pipeline97/1(d)
  [fifo0_re] -> pipeline101/1(d)
  pipeline130/1(q) -> fifo1/13(in_re)
  pipeline141/1(q) -> pipeline130/1(d)
  [fifo1_re] -> pipeline141/1(d)
  [hmc_sync] -> Gateway Out155/1, Counter/1
  Gateway Out155/1 -> To Workspace182/1
  [hmc_sync] -> FIFO1/4
  [hmc_sync] -> FIFO0/4
  [fifo0_empty] -> Gateway Out153/1, Inverter3/1
  [fifo1_empty] -> Gateway Out154/1, Inverter4/1
  Logical2/1 -> Counter19/2, delay2/1
  addr1/1 -> Gateway Out104/1, Relational/1, AddSub1/1
  [clear_hmc_addr_range] -> AddSub1/2
  AddSub1/1 -> Gateway Out156/1, Concat/1, Concat1/1
  Gateway Out156/1 -> To Workspace183/1
  Gateway Out157/1 -> To Workspace184/1
  Concat/1 -> Gateway Out157/1, [hmc_clear_wraddr_pol0]
  Gateway Out158/1 -> To Workspace185/1
  Constant6/1 -> Concat/2
  [hmc_reord_sync] -> delay4/1
  Shift/1 -> Gateway Out159/1, Gateway Out137/1, Relational/2
  Gateway Out159/1 -> To Workspace186/1
  edge_detect10/1(out) -> [fifo0_re]
  edge_detect28/1(out) -> [fifo1_re]
  [fifo0_empty] -> Inverter7/1
  [fifo1_empty] -> Inverter8/1
  [hmc_reord_data] -> Slice38/1, Slice37/1
  Gateway Out160/1 -> To Workspace187/1
  Mux7/1 -> Gateway Out164/1, Slice36/1
  Gateway Out161/1 -> To Workspace188/1
  Gateway Out162/1 -> To Workspace189/1
  Gateway Out163/1 -> To Workspace190/1
  [hmc_reord_dvalid] -> Register6/3, Register6/1, Gateway Out161/1, Mux7/1
  Slice36/1 -> [fifo_dout], Slice39/1, Gateway Out160/1
  Gateway Out164/1 -> To Workspace191/1
  Slice37/1 -> Gateway Out162/1, Mux7/2
  Slice38/1 -> Gateway Out163/1, Mux7/3
  Gateway Out165/1 -> To Workspace192/1
  [hmc_sync] -> Gateway Out166/1, Register6/2
  Gateway Out166/1 -> To Workspace193/1
  bus_expand16/2(out7) -> Gateway Out167/1
  bus_expand16/3(out6) -> Gateway Out168/1
  bus_expand16/4(out5) -> Gateway Out169/1
  bus_expand16/5(out4) -> Gateway Out170/1
  bus_expand16/6(out3) -> Gateway Out171/1
  bus_expand16/7(out2) -> Gateway Out172/1
  bus_expand16/8(lsb_out1) -> Gateway Out173/1
  Gateway Out173/1 -> To Workspace200/1
  Gateway Out172/1 -> To Workspace199/1
  Gateway Out171/1 -> To Workspace198/1
  Gateway Out170/1 -> To Workspace197/1
  Gateway Out169/1 -> To Workspace196/1
  Gateway Out168/1 -> To Workspace194/1
  Gateway Out167/1 -> To Workspace203/1
  bus_expand16/1(msb_out8) -> Gateway Out174/1
  Gateway Out174/1 -> To Workspace195/1
  Slice39/1 -> bus_expand16/1(bus_in)
  Mux/1 -> Terminator/1
  Register6/1 -> [fifo_dvalid], Gateway Out165/1
  Delay22/1 -> Delay9/1
  Gateway Out206/1 -> To Workspace232/1
  Slice43/1 -> bus_expand19/1(bus_in)
  bus_expand19/1(msb_out8) -> Gateway Out206/1
  Gateway Out191/1 -> To Workspace233/1
  Gateway Out192/1 -> To Workspace218/1
  Gateway Out193/1 -> To Workspace219/1
  bus_expand19/4(out5) -> Gateway Out193/1
  bus_expand19/3(out6) -> Gateway Out192/1
  bus_expand19/2(out7) -> Gateway Out191/1
  Gateway Out194/1 -> To Workspace220/1
  bus_expand19/5(out4) -> Gateway Out194/1
  Gateway Out195/1 -> To Workspace221/1
  bus_expand19/6(out3) -> Gateway Out195/1
  Gateway Out196/1 -> To Workspace222/1
  bus_expand19/7(out2) -> Gateway Out196/1
  Gateway Out197/1 -> To Workspace223/1
  bus_expand19/8(lsb_out1) -> Gateway Out197/1
  Slice42/1 -> bus_expand20/1(bus_in)
  Gateway Out198/1 -> To Workspace224/1
  Gateway Out199/1 -> To Workspace225/1
  Gateway Out200/1 -> To Workspace226/1
  Gateway Out201/1 -> To Workspace227/1
  Gateway Out202/1 -> To Workspace228/1
  Gateway Out203/1 -> To Workspace229/1
  Gateway Out204/1 -> To Workspace230/1
  Gateway Out205/1 -> To Workspace231/1
  bus_expand20/1(msb_out8) -> Gateway Out198/1
  bus_expand20/2(out7) -> Gateway Out199/1
  bus_expand20/3(out6) -> Gateway Out200/1
  bus_expand20/4(out5) -> Gateway Out201/1
  bus_expand20/5(out4) -> Gateway Out202/1
  bus_expand20/6(out3) -> Gateway Out203/1
  bus_expand20/7(out2) -> Gateway Out204/1
  bus_expand20/8(lsb_out1) -> Gateway Out205/1
  Delay23/1 -> Delay10/1
